simulink model "drive_cycle"  (R2023a)
settings: configuration reference "SharedConfig" (kept outside this file)
libraries: simulink x1
settings Model: Creator=frede  LastModifiedBy=ga84jar
settings ConfigSetRef: SourceName=SharedConfig  SourceLocation=Base Workspace

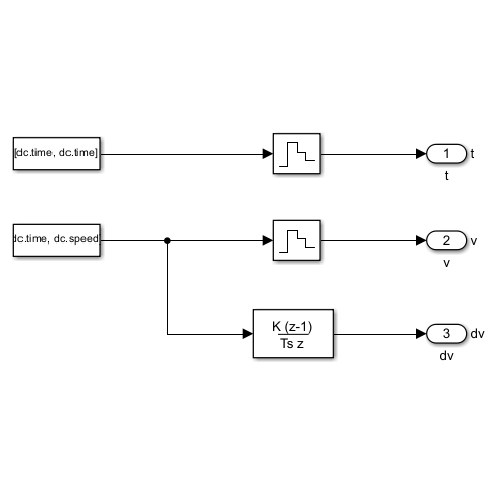
[thumbnail: Simulink's stored preview of the top-level diagram]
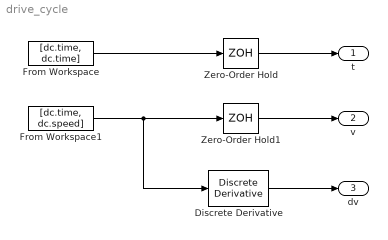
== system drive_cycle ==
  Discrete Derivative : simulink/Discrete/Discrete Derivative  gainval=1.0  ICPrevScaledInput=0.0  OutMin=[]  OutMax=[]  OutDataType=fixdt(1, 16)  OutScaling=2^-10  DoSatur=off
  From Workspace : FromWorkspace  VariableName=[dc.time, dc.time]
  From Workspace1 : FromWorkspace  VariableName=[dc.time, dc.speed]  OutputAfterFinalValue=Holding final value
  Zero-Order Hold : ZeroOrderHold  SampleTime=-1
  Zero-Order Hold1 : ZeroOrderHold  SampleTime=-1
  t : Outport  SignalName=t
  v : Outport  Port=2  SignalName=v
  dv : Outport  Port=3  SignalName=dv
  wires:
  Discrete Derivative/1 -> dv/1
  From Workspace/1 -> Zero-Order Hold/1
  From Workspace1/1 -> Zero-Order Hold1/1, Discrete Derivative/1
  Zero-Order Hold/1 -> t/1
  Zero-Order Hold1/1 -> v/1
